simulink model "Pole_Placement_Continuous"  (Simulink 8.9)
settings: Solver=VariableStepAuto  StartTime=0.0  StopTime=60  RelTol=1e-3
values from neighbouring files (symbols this model uses):
  f0 = F(2)    [Lab3_Pole_Placement.m]
  f1 = F(1)    [Lab3_Pole_Placement.m]
  g0 = F(4)    [Lab3_Pole_Placement.m]
  g1 = F(3)    [Lab3_Pole_Placement.m]
  K1 = 0.66538    [Lab3_Pole_Placement.m]
  K2 = 0.062    [Lab3_Pole_Placement.m]
  K3 = 4.78    [Lab3_Pole_Placement.m]
  Kp = 15    [Lab3_Pole_Placement.m]
  Kp_c2 = 1 / DC_gain    [Lab3_Pole_Placement.m]
  p = 10.5    [Lab3_Pole_Placement.m]
  tau = 0.030541    [Lab3_Pole_Placement.m]
  z = 10    [Lab3_Pole_Placement.m]
settings Model: Creator=joe  LastModifiedBy=joe
settings DataIOCC: LimitDataPoints=off  SaveFormat=Dataset  SignalLoggingSaveFormat=Dataset
settings DebuggingCC: UnderspecifiedInitializationDetection=Simplified  MergeDetectMultiDrivingBlocksExec=error  FcnCallInpInsideContextMsg=error  StateNameClashWarn=none  SFUnexpectedBacktrackingDiag=error  SFNoUnconditionalDefaultTransitionDiag=error
settings HardwareCC: ProdBitPerPointer=64  ProdBitPerSizeT=64  ProdBitPerPtrDiffT=64  ProdLargestAtomicFloat=Float  ProdIntDivRoundTo=Zero  ProdEndianess=LittleEndian  ProdWordSize=64  ProdHWDeviceType=Intel->x86-64 (Windows64)
settings ModelReferenceCC: PropagateSignalLabelsOutOfModel=on
settings GRTTargetCC: TargetLangStandard=C99 (ISO)  GeneratePreprocessorConditionals=Use local settings  CombineOutputUpdateFcns=on  GRTInterface=off
settings ConfigComp: CovMetricSettings=dwe  CovHtmlReporting=off  CovSaveCumulativeToWorkspaceVar=off  CovSaveSingleToWorkspaceVar=off  CovExternalEMLEnable=on

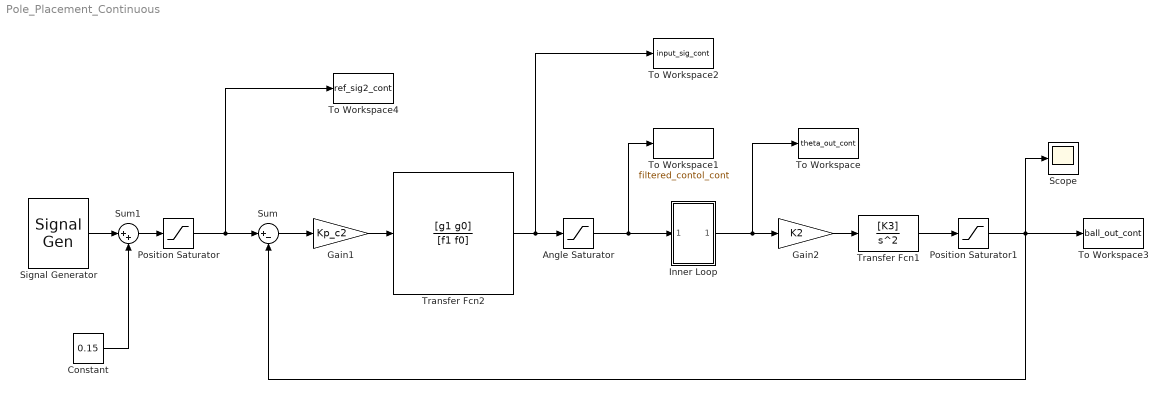
== system Pole_Placement_Continuous ==
  Angle Saturator : Saturate  UpperLimit=0.785  LowerLimit=-0.785
  Constant : Constant  Value=0.15
  Gain1 : Gain  Gain=Kp_c2
  Gain2 : Gain  Gain=K2
  Inner Loop : Subsystem
  Position Saturator : Saturate  UpperLimit=0.417  LowerLimit=0
  Position Saturator1 : Saturate  UpperLimit=0.417  LowerLimit=0
  Scope : Scope
  Signal Generator : SignalGenerator  WaveForm=square  Amplitude=0.03  Frequency=0.05
  Sum : Sum  Inputs=|+-
  Sum1 : Sum  Inputs=|++
  To Workspace : ToWorkspace  VariableName=theta_out_cont  SaveFormat=Timeseries  SampleTime=-1
  To Workspace1 : ToWorkspace  VariableName=filtered_contol_cont  SaveFormat=Timeseries  SampleTime=-1
  To Workspace2 : ToWorkspace  VariableName=input_sig_cont  SaveFormat=Timeseries  SampleTime=-1
  To Workspace3 : ToWorkspace  VariableName=ball_out_cont  SaveFormat=Timeseries  SampleTime=-1
  To Workspace4 : ToWorkspace  VariableName=ref_sig2_cont  SaveFormat=Timeseries  SampleTime=-1
  Transfer Fcn1 : TransferFcn  Numerator=[K3]  Denominator=[1 0 0]
  Transfer Fcn2 : TransferFcn  Numerator=[g1 g0]  Denominator=[f1 f0]
  wires:
  Transfer Fcn2/1 -> To Workspace2/1, Angle Saturator/1
  Angle Saturator/1 -> To Workspace1/1, Inner Loop/1(In1)
  Gain1/1 -> Transfer Fcn2/1
  Sum/1 -> Gain1/1
  Position Saturator/1 -> To Workspace4/1, Sum/1
  Gain2/1 -> Transfer Fcn1/1
  Inner Loop/1(Out1) -> To Workspace/1, Gain2/1
  Transfer Fcn1/1 -> Position Saturator1/1
  Position Saturator1/1 -> Scope/1, To Workspace3/1, Sum/2
  Constant/1 -> Sum1/2
  Signal Generator/1 -> Sum1/1
  Sum1/1 -> Position Saturator/1

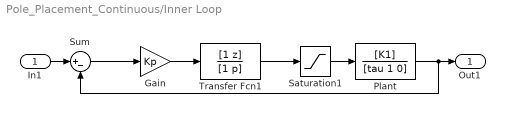
== system Pole_Placement_Continuous/Inner Loop ==
  In1 : Inport
  Gain : Gain  Gain=Kp
  Plant : TransferFcn  Numerator=[K1]  Denominator=[tau 1 0]
  Saturation1 : Saturate  UpperLimit=6  LowerLimit=-6
  Sum : Sum  Inputs=|+-
  Transfer Fcn1 : TransferFcn  Numerator=[1 z]  Denominator=[1 p]
  Out1 : Outport
  wires:
  In1/1 -> Sum/1
  Plant/1 -> Sum/2, Out1/1
  Gain/1 -> Transfer Fcn1/1
  Transfer Fcn1/1 -> Saturation1/1
  Sum/1 -> Gain/1
  Saturation1/1 -> Plant/1
